simulink model "autosar_bsw_inject"  (R2022b)
settings: Solver=FixedStepAuto  StartTime=0.0  StopTime=10.0  FixedStep=0.1  RelTol=1e-3
undefined symbols (not defined in the file): Dem_EventStatusType
libraries: simulink x3, autosarlibdem x3
settings Model: Creator=The MathWorks, Inc.  LastModifiedBy=The MathWorks, Inc.
settings SolverCC: MaxZcPerStep=1
settings OptimizationCC: DefaultParameterBehavior=Inlined  EnhancedBackFolding=on  PassReuseOutputArgsAs=Individual arguments  ZeroExternalMemoryAtStartup=off  ZeroInternalMemoryAtStartup=off  OptimizeBlockOrder=speed  DifferentSizesBufferReuse=on  OptimizationCustomize=off  EfficientTunableParamExpr=on
settings DebuggingCC: ParameterTunabilityLossMsg=error
settings ModelReferenceCC: EnableRefExpFcnMdlSchedulingChecks=on
settings SFSimCC: MATLABDynamicMemAlloc=off
settings RTWCC: Description=AUTOSAR  SystemTargetFile=autosar.tlc  GenCodeOnly=on  TemplateMakefile=ert_default_tmf  DLArmComputeVersion=19.05
settings CodeAppCC: ForceParamTrailComments=on  IgnoreCustomStorageClasses=off  OperatorAnnotations=on  SimulinkDataObjDesc=on  SFDataObjDesc=on  InsertBlockDesc=on
settings STFCustomTargetCC: TargetLangStandard=C99 (ISO)  MultiwordLength=256  ParMdlRefBuildCompliant=on  CompOptLevelCompliant=on  IncludeMdlTerminateFcn=off  CombineOutputUpdateFcns=on  SuppressErrorStatus=on  ERTCustomFileBanners=on  SupportNonFinite=off  SupportComplex=off  SupportContinuousTime=off  SupportNonInlinedSFcns=off  RemoveResetFunc=on  MATLABClassNameForMDSCustomization=Simulink.SoftwareTarget.ERTCustomization  AutosarCompliant=on  UseToolchainInfoCompliant=on  LookupTableObjectStructAxisOrder=2,1,3,4,...  LUTObjectStructOrderEvenSpacing=Size,Table,Breakpoints  SystemTargetFile=autosar.tlc
settings ERTTargetCC: TargetLangStandard=C99 (ISO)  ConcurrentExecutionCompliant=off  IncludeMdlTerminateFcn=off  SuppressErrorStatus=on  SupportNonFinite=off  SupportComplex=off  ModelStepFunctionPrototypeControlCompliant=off  CPPClassGenCompliant=off  AutosarCompliant=on  LookupTableObjectStructAxisOrder=2,1,3,4,...  LUTObjectStructOrderEvenSpacing=Size,Table,Breakpoints  InlinedParameterPlacement=NonHierarchical  ERTCustomFileTemplate=example_file_process.tlc

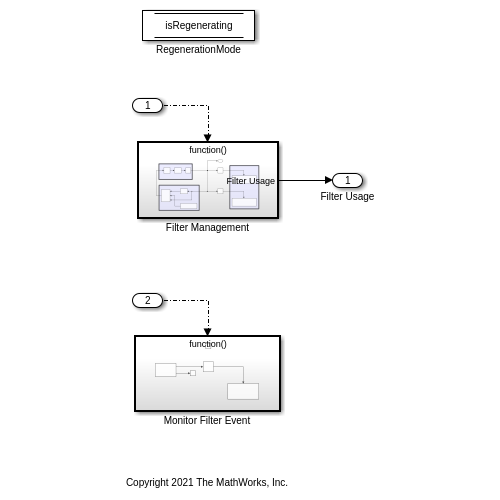
[thumbnail: Simulink's stored preview of the top-level diagram]
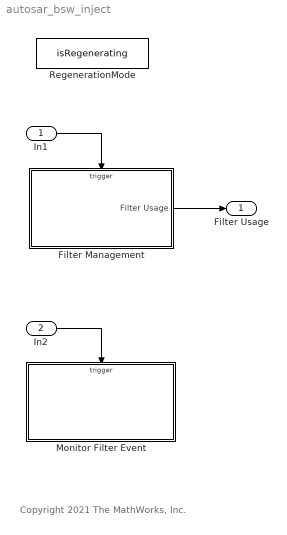
== system autosar_bsw_inject ==
  note: Copyright 2021 The MathWorks, Inc.
  In1 : Inport  SampleTime=0.1  OutputFunctionCall=on
  In2 : Inport  Port=2  SampleTime=0.1  OutputFunctionCall=on
  Filter Management : Subsystem
  Monitor Filter Event : Subsystem
  RegenerationMode : DataStoreMemory  DataStoreName=isRegenerating  InitialValue=false  ShowAdditionalParam=off  OutDataTypeStr=boolean
  Filter Usage : Outport
  wires:
  Filter Management/1(Filter Usage) -> Filter Usage/1
  In1/1 -> Filter Management/Trigger
  In2/1 -> Monitor Filter Event/Trigger

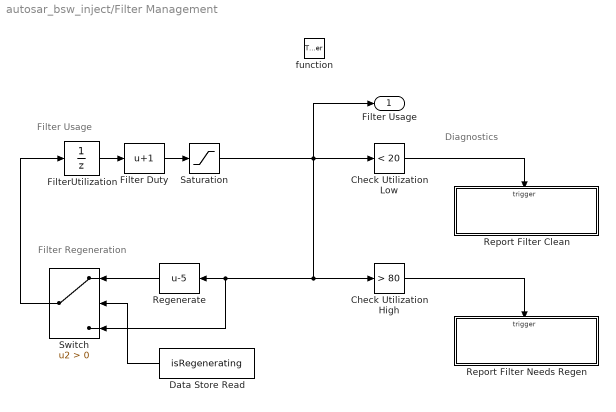
== system autosar_bsw_inject/Filter Management ==
  note: Diagnostics
  note: Filter Usage
  note: Filter Regeneration
  function : TriggerPort  TriggerType=function-call  VariantControl=(inherit)
  Check Utilization High : simulink/Logic and Bit Operations/Compare To Constant  relop=>  const=80  OutDataTypeStr=boolean
  Check Utilization Low : simulink/Logic and Bit Operations/Compare To Constant  relop=<  const=20  OutDataTypeStr=boolean
  Data Store Read : DataStoreRead  DataStoreName=isRegenerating  IndexOptions=Index vector (dialog)  Indices=1  OutputSizes=1
  Filter Duty : Bias  Bias=1  SaturateOnIntegerOverflow=off
  FilterUtilization : UnitDelay  InitialCondition=50  SampleTime=-1  HasFrameUpgradeWarning=on
      settings: AttributesFormatString=Initial Value: %<InitialCondition>
  Regenerate : Bias  Bias=-5  SaturateOnIntegerOverflow=off
  Report Filter Clean : Subsystem
  Report Filter Needs Regen : Subsystem
  Saturation : Saturate  UpperLimit=100  LowerLimit=0
  Switch : Switch  Criteria=u2 > Threshold  SaturateOnIntegerOverflow=off  InputSameDT=off
  Filter Usage : Outport
  wires:
  Switch/1 -> FilterUtilization/1
  FilterUtilization/1 -> Filter Duty/1
  Check Utilization Low/1 -> Report Filter Clean/Trigger
  Filter Duty/1 -> Saturation/1
  Saturation/1 -> Filter Usage/1, Regenerate/1, Switch/3, Check Utilization High/1, Check Utilization Low/1
  Check Utilization High/1 -> Report Filter Needs Regen/Trigger
  Data Store Read/1 -> Switch/2
  Regenerate/1 -> Switch/1

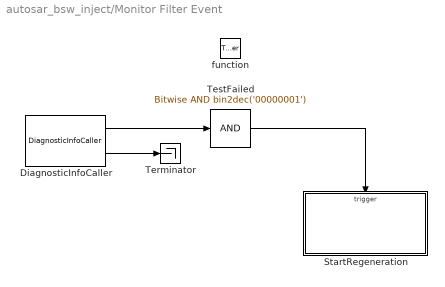
== system autosar_bsw_inject/Monitor Filter Event ==
  function : TriggerPort  TriggerType=function-call  VariantControl=(inherit)
  DiagnosticInfoCaller : autosarlibdem/DiagnosticInfoCaller  PortName=FilterInfo  Operation=GetEventStatus  st=-1  ServiceImpl=autosar.bsw.DemDiagnosticInfo
  StartRegeneration : Subsystem
  Terminator : Terminator
  TestFailed : simulink/Logic and Bit Operations/Bitwise Operator  logicop=AND  UseBitMask=on  BitMask=bin2dec('00000001')  BitMaskRealWorld=Stored Integer
  wires:
  TestFailed/1 -> StartRegeneration/Trigger
  DiagnosticInfoCaller/2 -> Terminator/1
  DiagnosticInfoCaller/1 -> TestFailed/1

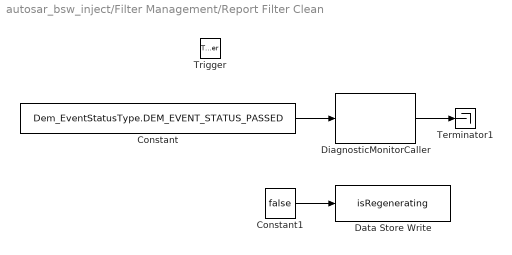
== system autosar_bsw_inject/Filter Management/Report Filter Clean ==
  Trigger : TriggerPort  VariantControl=(inherit)  PortDimensions=1
  Constant : Constant  Value=Dem_EventStatusType.DEM_EVENT_STATUS_PASSED
  Constant1 : Constant  Value=false
  Data Store Write : DataStoreWrite  DataStoreName=isRegenerating  IndexOptions=Index vector (dialog)  Indices=1  OutputSizes=1
  DiagnosticMonitorCaller : autosarlibdem/DiagnosticMonitorCaller  PortName=FilterMonitor  Operation=SetEventStatus  Datatype=Enum: Dem_EventStatusType  st=-1  ServiceImpl=autosar.bsw.DemDiagnosticMonitor
  Terminator1 : Terminator
  wires:
  Constant/1 -> DiagnosticMonitorCaller/1
  DiagnosticMonitorCaller/1 -> Terminator1/1
  Constant1/1 -> Data Store Write/1

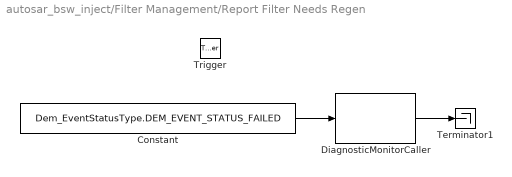
== system autosar_bsw_inject/Filter Management/Report Filter Needs Regen ==
  Trigger : TriggerPort  VariantControl=(inherit)  PortDimensions=1
  Constant : Constant  Value=Dem_EventStatusType.DEM_EVENT_STATUS_FAILED
  DiagnosticMonitorCaller : autosarlibdem/DiagnosticMonitorCaller  PortName=FilterMonitor  Operation=SetEventStatus  Datatype=Enum: Dem_EventStatusType  st=-1  ServiceImpl=autosar.bsw.DemDiagnosticMonitor
  Terminator1 : Terminator
  wires:
  DiagnosticMonitorCaller/1 -> Terminator1/1
  Constant/1 -> DiagnosticMonitorCaller/1

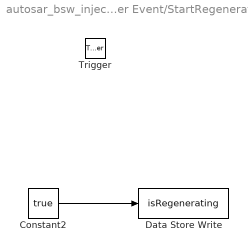
== system autosar_bsw_inject/Monitor Filter Event/StartRegeneration ==
  Trigger : TriggerPort  VariantControl=(inherit)  PortDimensions=1
  Constant2 : Constant  Value=true
  Data Store Write : DataStoreWrite  DataStoreName=isRegenerating  IndexOptions=Index vector (dialog)  Indices=1  OutputSizes=1
  wires:
  Constant2/1 -> Data Store Write/1
